simulink model "mcb_open_loop_control_nucleo_f401re"  (R2024b)
settings: Solver=FixedStepDiscrete  StartTime=0.0  StopTime=inf  RelTol=1e-3  EnableMultiTasking=on
InitFcn:
  | mcb_open_loop_control_data;
  | 
  | target.model                = 'NUCLEO-F446RE';	  % 	// Manufacturer Model Number
  | target.sn                   = 'xx';          	  % 	// Manufacturer Serial Number
  | target.CPU_frequency        = 84e6;    		  %Hz  // Clock frequency
  | target.PWM_frequency        = PWM_frequency;   	  %Hz  // PWM frequency
  | target.PWM_Counter_Period   = ...
  |  round(target.CPU_frequency/target.PWM_frequency/2); %    //PWM timer counts for up-down counter
  | target.ADC_Vref             = 3.3;			  %V   // ADC voltage reference for NUCLEO-F401RE
  | target.ADC_MaxCount         = 4095;			  %    // Max count for 12 bit ADC
  | %Read inverter logic from 'Configuration' panel on model
  | inverter.EnableLogic = eval(get_param([bdroot '/Open Loop Control/Parameters/Inverter'],'Value'));
model workspace (MAT data in the model file):
  MaxVsecuryte = 200
undefined symbols (not defined in the file or in its folder): DiscIntNeverNeededParam, motor, Ts
libraries: stmutilitieslib x4, stm32f4xxblockslib x4, simulink x3, mcbcontrolslib x3, stm32blockslib x2, hdlsllib x1, canmsglib x1
settings Model: STM32="{\"DigitalPortWrite\":{\"ID\":\"mcb_open_loop_control_nucleo_f401re:3779\"},\"PWMOutput\":{\"ID\":\"mcb_open_loop_control_nucleo_f401re:3778\"},\"HardwareInterrupt\":{\"ID\":\"mcb_open_loop_control_nucleo_f401re:3773\"},\"AnalogInput\":{\"ID\":\"mcb_open_loop_control_nucleo_f401re:3774\"},\"CANWrite\":{\"ID\":\"mcb_open_loop_control_nucleo_f401re:3906\"},\"CANRead\":{\"ID\":\"mcb_open_loop_control_nucleo_f401re:3916\"}}"  CodeVerificationMode=processor-in-the-loop (pil)  Creator=The MathWorks, Inc.  LastModifiedBy=aferreira
settings SolverCC: AlgebraicLoopSolver=TrustRegion  AutoInsertRateTranBlk=on  MaxZcPerStep=1
settings DataIOCC: SaveOutput=off  SaveTime=off  ReturnWorkspaceOutputs=off
settings OptimizationCC: DefaultUnderspecifiedDataType=single  EnhancedBackFolding=on  PassReuseOutputArgsAs=Individual arguments  ZeroExternalMemoryAtStartup=off  EfficientFloat2IntCast=on  MaxStackSize=512  OptimizeBlockOrder=speed  DifferentSizesBufferReuse=on  OptimizationCustomize=off  EfficientTunableParamExpr=on
settings DebuggingCC: MultiTaskDSMMsg=none  ParameterPrecisionLossMsg=none  ParameterTunabilityLossMsg=error  UnconnectedInputMsg=warning  UnconnectedOutputMsg=warning  UnconnectedLineMsg=warning  SubsystemReferenceDiagnosticForUnitTest=warning
settings HardwareCC: ProdBitPerPointer=32  ProdBitPerSizeT=32  ProdBitPerPtrDiffT=32  ProdLargestAtomicInteger=Long  ProdLargestAtomicFloat=Double  ProdWordSize=32  ProdLongLongMode=on  ProdHWDeviceType=ARM Compatible->ARM Cortex
settings ModelReferenceCC: EnableRefExpFcnMdlSchedulingChecks=on
settings SFSimCC: MATLABDynamicMemAlloc=off
settings RTWCC: Description=Embedded Coder  SystemTargetFile=ert.tlc  HardwareBoard=STM32F4xx Based  TemplateMakefile=ert_default_tmf  GenerateReport=on  Toolchain=GNU Tools for ARM Embedded Processors  BuildConfiguration=Faster Runs  IncludeHyperlinkInReport=on  CodeProfilingSaveOptions=AllData  GenerateTraceInfo=on  GenerateTraceReport=on  GenerateTraceReportSl=on  GenerateTraceReportSf=on  GenerateTraceReportEml=on  GPUComputeCapability=3.5  DLArmComputeVersion=19.05
settings CodeAppCC: ForceParamTrailComments=on  IgnoreCustomStorageClasses=off  OperatorAnnotations=on  SimulinkDataObjDesc=on  SFDataObjDesc=on  InsertBlockDesc=on
settings ERTTargetCC: TargetLangStandard=C99 (ISO)  CodeReplacementLibrary=ARM Cortex-M  ExtModeTransport=3  ExtModeStaticAlloc=on  ExtModeStaticAllocSize=16384  ExtModeMexFile=ext_xcp  ExtModeIntrfLevel=Level2 - Open  InlinedParameterPlacement=Hierarchical  DynamicArrayContainerType=coder::array

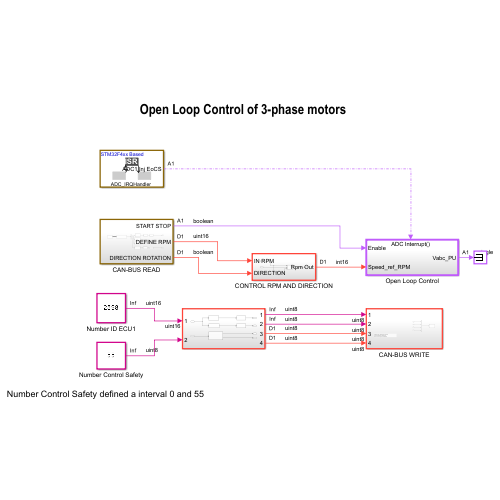
[thumbnail: Simulink's stored preview of the top-level diagram]
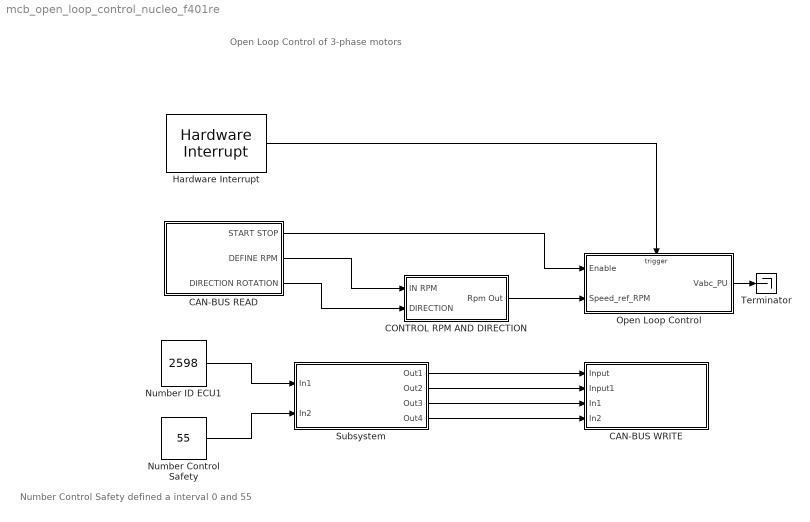
== system mcb_open_loop_control_nucleo_f401re ==
  note: Open Loop Control of 3-phase motors
  note: Number Control Safety defined a interval 0 and 55
  CAN-BUS READ : Subsystem
  CAN-BUS WRITE : Subsystem
  CONTROL RPM AND DIRECTION : Subsystem
  Hardware Interrupt : stm32f4xxblockslib/Hardware Interrupt  ISRGroup=Analog to digital converter (ADC)  ISRName=ADC_IRQHandler  ISRNumber=33  EventsList={ 'off', 'ADC1 OVR', '1'; 'off', 'ADC1 Reg EoCS', '2'; 'on', 'ADC1 Inj EoCS', '3'; 'off', 'ADC1 Watchdog', '4'; 'off', 'ADC2 OVR', '5'; 'off', 'ADC2 Reg EoCS', '6'; 'off', 'ADC2 Inj EoCS', '7'; 'off', 'ADC2 Watchdog', '8'; 'off', 'ADC3 OVR', '9'; 'off', 'ADC3 Reg EoCS', '10'; 'off', 'ADC3 Inj EoCS', '11'; 'off', 'ADC3 Watchdog', '12'; 'off', 'Custom event', '13' }  SelectedEvents={'ADC1 Inj EoCS'}  TaskPriority=30  DisablePreemption=off  ClearInterruptFlagsAtEndOfEvent=off  InterruptDefinitionFile=$(TARGET_ROOT)/registry/interrupts/STM32F4xxBased_interrupts.xml  HardwareBoard=STM32F4xx Based  EnableSimPort=off
  Number Control Safety : Constant  Value=55  OutMin=0  OutMax=55  OutDataTypeStr=uint8
  Number ID ECU1 : Constant  Value=2598  OutDataTypeStr=uint16
  Open Loop Control : Subsystem
  Subsystem : Subsystem
  Terminator : Terminator
  wires:
  Open Loop Control/1(Vabc_PU) -> Terminator/1
  Hardware Interrupt/1 -> Open Loop Control/Trigger
  CAN-BUS READ/2(DEFINE RPM) -> CONTROL RPM AND DIRECTION/1(IN RPM)
  CAN-BUS READ/3(DIRECTION ROTATION) -> CONTROL RPM AND DIRECTION/2(DIRECTION)
  CONTROL RPM AND DIRECTION/1(Rpm Out) -> Open Loop Control/2(Speed_ref_RPM)
  CAN-BUS READ/1(START STOP) -> Open Loop Control/1(Enable)
  Number ID ECU1/1 -> Subsystem/1(In1)
  Number Control Safety/1 -> Subsystem/2(In2)
  Subsystem/1(Out1) -> CAN-BUS WRITE/1(Input)
  Subsystem/2(Out2) -> CAN-BUS WRITE/2(Input1)
  Subsystem/3(Out3) -> CAN-BUS WRITE/3(In1)
  Subsystem/4(Out4) -> CAN-BUS WRITE/4(In2)

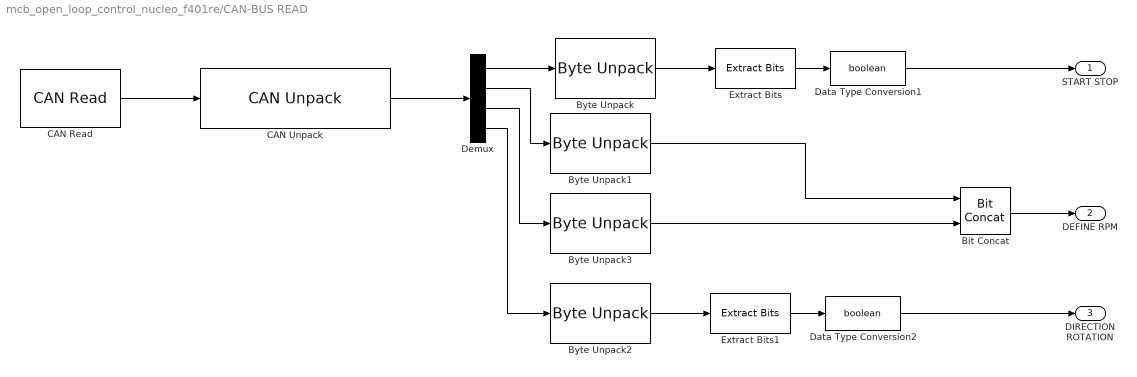
== system mcb_open_loop_control_nucleo_f401re/CAN-BUS READ ==
  Bit Concat : hdlsllib/Logic and Bit Operations/Bit Concat  numInputs=2
  Byte Unpack{,1..3} (4 alike) : stmutilitieslib/Byte Unpack  dimensions={[1]}  datatypes={'uint8'}  byteAlign=1  blockPlatform=stm32f4discovery
  CAN Read : stm32blockslib/CAN Read  CANModule=CAN1  BlockMode=Receive  OperationReadMode=Data  OperationWriteMode=Data  OutputTypeReadMode=Packed  DataFormatWriteMode=Raw data  ReadSource=FIFO 0  IdentifierTypeVia=Dialog  IdentifierType=Standard (11-bit identifier)  IdentifierVia=Inport  Identifier=100  DataLengthVia=Inport  DataLength=8  OutputIdType=off  TransmitRemoteFrame=off  OutputRemoteFrame=off  OutputTxFifoLevel=off  OutputRxFifoLevel=off  OutputStatus=off  Timeout=0.001  SampleTime=-1
      settings: LibrarySourceBlock=stm32f4xxblockslib/CAN Read
  CAN Unpack : canmsglib/CAN Unpack  MsgList=(none)  MsgName=CAN Msg  MsgIDType=Standard (11-bit identifier)  MsgIdentifier=0x220  MsgLength=4  SignalInfo={}  IDPort=off  TimestampPort=off  ErrorPort=off  RemotePort=off  LengthPort=off  StatusPort=off  ApplyMinMax=off
      settings: LibrarySourceBlock=stmutilitieslib/CAN Unpack  DataFormat=raw data
  Data Type Conversion1 : DataTypeConversion  OutDataTypeStr=boolean  SaturateOnIntegerOverflow=off  RndMeth=Floor
  Data Type Conversion2 : DataTypeConversion  OutDataTypeStr=boolean  SaturateOnIntegerOverflow=off  RndMeth=Floor
  Demux : Demux
  Extract Bits : simulink/Logic and Bit Operations/Extract Bits  bitsToExtract=Range of bits  numBits=8  bitIdxRange=[0]  outScalingMode=Preserve fixed-point scaling
  Extract Bits1 : simulink/Logic and Bit Operations/Extract Bits  bitsToExtract=Range of bits  numBits=8  bitIdxRange=[0]  outScalingMode=Preserve fixed-point scaling
  START STOP : Outport
  DEFINE RPM : Outport  Port=2
  DIRECTION ROTATION : Outport  Port=3
  wires:
  CAN Unpack/1 -> Demux/1
  Demux/1 -> Byte Unpack/1
  Data Type Conversion1/1 -> START STOP/1
  Byte Unpack/1 -> Extract Bits/1
  CAN Read/1 -> CAN Unpack/1
  Demux/2 -> Byte Unpack1/1
  Extract Bits/1 -> Data Type Conversion1/1
  Extract Bits1/1 -> Data Type Conversion2/1
  Data Type Conversion2/1 -> DIRECTION ROTATION/1
  Byte Unpack2/1 -> Extract Bits1/1
  Demux/3 -> Byte Unpack3/1
  Demux/4 -> Byte Unpack2/1
  Bit Concat/1 -> DEFINE RPM/1
  Byte Unpack1/1 -> Bit Concat/1
  Byte Unpack3/1 -> Bit Concat/2

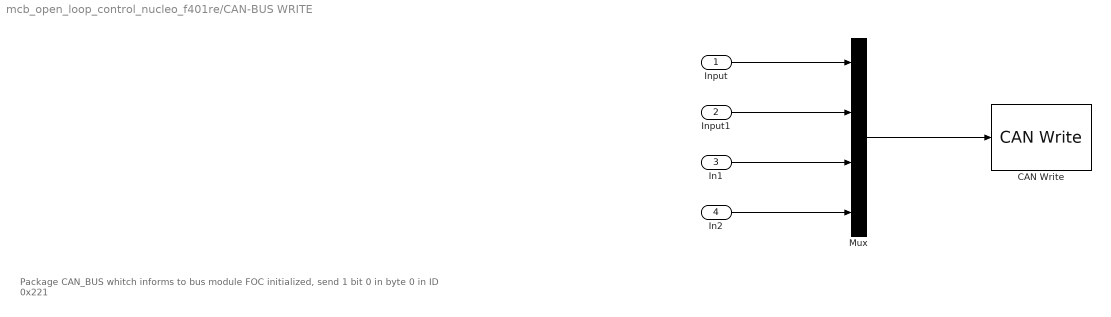
== system mcb_open_loop_control_nucleo_f401re/CAN-BUS WRITE ==
  note: Package CAN_BUS whitch informs
      | to bus module FOC initialized,
      | send 1 bit 0 in byte 0 in ID 0x221
  Input : Inport  OutDataTypeStr=uint8
  Input1 : Inport  Port=2  OutDataTypeStr=uint8
  In1 : Inport  Port=3  OutDataTypeStr=uint8
  In2 : Inport  Port=4  OutDataTypeStr=uint8
  CAN Write : stm32blockslib/CAN Write  CANModule=CAN1  BlockMode=Transmit  OperationReadMode=Data  OperationWriteMode=Data  OutputTypeReadMode=Unpacked  DataFormatWriteMode=Raw data  ReadSource=FIFO 0  IdentifierTypeVia=Dialog  IdentifierType=Standard (11-bit identifier)  IdentifierVia=Dialog  Identifier=0x221  DataLengthVia=Dialog  DataLength=4  OutputIdType=off  TransmitRemoteFrame=off  OutputRemoteFrame=off  OutputTxFifoLevel=off  OutputRxFifoLevel=off  OutputStatus=off  Timeout=0.1  SampleTime=-1
      settings: LibrarySourceBlock=stm32f4xxblockslib/CAN Write
  Mux : Mux
  wires:
  Mux/1 -> CAN Write/1
  Input/1 -> Mux/1
  Input1/1 -> Mux/2
  In1/1 -> Mux/3
  In2/1 -> Mux/4

== system mcb_open_loop_control_nucleo_f401re/CONTROL RPM AND DIRECTION ==
  IN RPM : Inport
  DIRECTION : Inport  Port=2
  Gain : Gain  Gain=-1  ParamDataTypeStr=int16  OutDataTypeStr=int16  RndMeth=Simplest
  Switch : Switch  Criteria=u2 ~= 0  OutDataTypeStr=int16  RndMeth=Simplest  SaturateOnIntegerOverflow=off  InputSameDT=off
  Rpm Out : Outport
  wires:
  Switch/1 -> Rpm Out/1
  IN RPM/1 -> Gain/1, Switch/1
  DIRECTION/1 -> Switch/2
  Gain/1 -> Switch/3

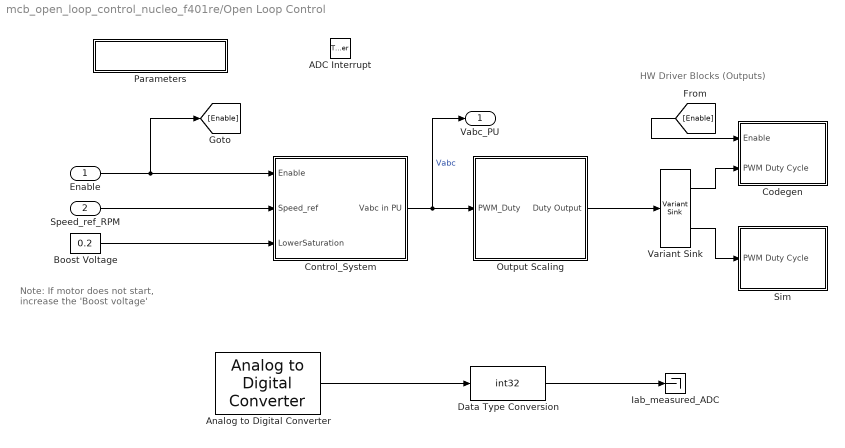
== system mcb_open_loop_control_nucleo_f401re/Open Loop Control ==
  note: Note: If motor does not start, increase the 'Boost voltage'
  note: HW Driver Blocks (Outputs)
  Enable : Inport
  Speed_ref_RPM : Inport  Port=2
  ADC Interrupt : TriggerPort  TriggerType=function-call  VariantControl=Variant
  Analog to Digital Converter : stm32f4xxblockslib/Analog to Digital Converter  ADCModule=ADC1  ConversionGroup=Injected  TriggerMode=Read results only  NumberOfConversions=2  EnableBufferConv=off  BufferLength=1  OutputStatus=off  SampleTime=-1  EnableSimPort=off  hoistedMaskSrc=ECSoC/ECSimCodegen/Analog to Digital Converter
  Boost Voltage : Constant  Value=0.2  OutDataTypeStr=dataType
  Codegen : Subsystem
      settings: RTWSystemCode=Nonreusable function
  Control_System : Subsystem
      settings: RTWSystemCode=Nonreusable function
  Data Type Conversion : DataTypeConversion  OutDataTypeStr=int32  ConvertRealWorld=Stored Integer (SI)  SaturateOnIntegerOverflow=off  RndMeth=Floor
  Iab_measured_ADC : Terminator
  Output Scaling : Subsystem
      settings: RTWSystemCode=Nonreusable function
  Parameters : Subsystem
  Sim : Subsystem
  Variant Sink : VariantSink  VariantControlMode=sim codegen switching
  Vabc_PU : Outport  VectorParamsAs1DForOutWhenUnconnected=off
  wires:
  Control_System/1(Vabc in PU) -> Output Scaling/1(PWM_Duty), Vabc_PU/1  "Vabc"
  Boost Voltage/1 -> Control_System/3(LowerSaturation)
  Data Type Conversion/1 -> Iab_measured_ADC/1
  Enable/1 -> [Enable], Control_System/1(Enable)
  Speed_ref_RPM/1 -> Control_System/2(Speed_ref)
  Analog to Digital Converter/1 -> Data Type Conversion/1
  [Enable] -> Codegen/1(Enable)
  Variant Sink/1 -> Codegen/2(PWM Duty Cycle)
  Variant Sink/2 -> Sim/1(PWM Duty Cycle)
  Output Scaling/1(Duty Output) -> Variant Sink/1

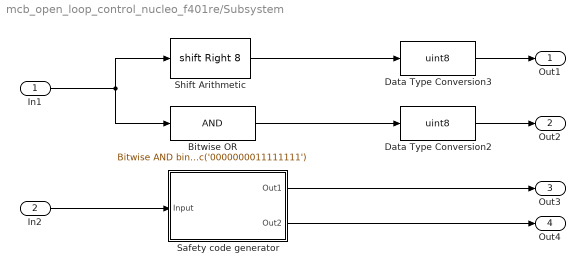
== system mcb_open_loop_control_nucleo_f401re/Subsystem ==
  In1 : Inport  OutDataTypeStr=uint16
  In2 : Inport  Port=2
  Bitwise OR : simulink/Logic and Bit Operations/Bitwise Operator  logicop=AND  UseBitMask=on  BitMask=bin2dec('0000000011111111')  BitMaskRealWorld=Stored Integer
  Data Type Conversion2 : DataTypeConversion  OutDataTypeStr=uint8  SaturateOnIntegerOverflow=off  RndMeth=Floor
  Data Type Conversion3 : DataTypeConversion  OutDataTypeStr=uint8  SaturateOnIntegerOverflow=off  RndMeth=Floor
  Safety code generator : Subsystem
  Shift Arithmetic : ArithShift  BitShiftNumber=8  BitShiftDirection=Right
  Out1 : Outport  OutDataTypeStr=uint8
  Out2 : Outport  Port=2  OutDataTypeStr=uint8
  Out3 : Outport  Port=3  OutDataTypeStr=uint8
  Out4 : Outport  Port=4  OutDataTypeStr=uint8
  wires:
  Data Type Conversion3/1 -> Out1/1
  In2/1 -> Safety code generator/1(Input)
  Data Type Conversion2/1 -> Out2/1
  Safety code generator/2(Out2) -> Out4/1
  Safety code generator/1(Out1) -> Out3/1
  Bitwise OR/1 -> Data Type Conversion2/1
  In1/1 -> Bitwise OR/1, Shift Arithmetic/1
  Shift Arithmetic/1 -> Data Type Conversion3/1

== system mcb_open_loop_control_nucleo_f401re/Open Loop Control/Codegen ==
  Enable : Inport
  PWM Duty Cycle : Inport  Port=2
  Hardware Initialization : Subsystem
      settings: RTWSystemCode=Nonreusable function
  PWM Output : Subsystem
      settings: RTWSystemCode=Nonreusable function
  wires:
  PWM Duty Cycle/1 -> PWM Output/1(PWM Duty Cycle)
  Enable/1 -> Hardware Initialization/1(Enable), PWM Output/2(Enable)

== system mcb_open_loop_control_nucleo_f401re/Open Loop Control/Control_System ==
  Enable : Inport
  Speed_ref : Inport  Port=2
  LowerSaturation : Inport  Port=3
  SpeedRefToFreq : Subsystem
  VabcCalc : Subsystem
  Vabc in PU : Outport  VectorParamsAs1DForOutWhenUnconnected=off
  wires:
  Speed_ref/1 -> SpeedRefToFreq/2(Speed_Ref)
  SpeedRefToFreq/1(Frequency) -> VabcCalc/1(Frequency)
  VabcCalc/1(Vabc) -> Vabc in PU/1
  LowerSaturation/1 -> VabcCalc/2(LowerSaturation)
  Enable/1 -> SpeedRefToFreq/1(Enable)

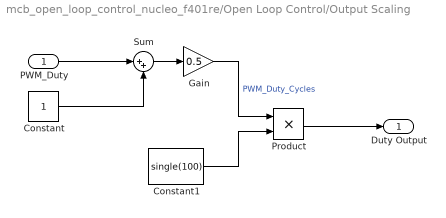
== system mcb_open_loop_control_nucleo_f401re/Open Loop Control/Output Scaling ==
  PWM_Duty : Inport
  Constant : Constant  OutDataTypeStr=dataType
  Constant1 : Constant  Value=single(100)
  Gain : Gain  Gain=0.5  RndMeth=Simplest  OutDataTypeStr=Inherit: Same as input
  Product : Product  RndMeth=Simplest  OutDataTypeStr=Inherit: Same as first input
  Sum : Sum  Inputs=|++
  Duty Output : Outport
  wires:
  Product/1 -> Duty Output/1
  Constant1/1 -> Product/2
  PWM_Duty/1 -> Sum/1
  Constant/1 -> Sum/2
  Sum/1 -> Gain/1
  Gain/1 -> Product/1  "PWM_Duty_Cycles"

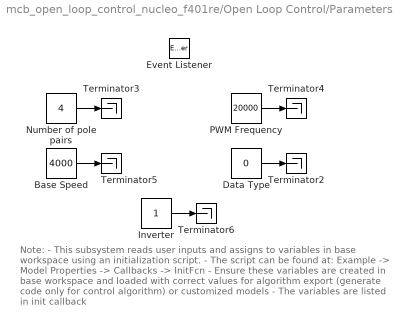
== system mcb_open_loop_control_nucleo_f401re/Open Loop Control/Parameters ==
  note: Note:
      | - This subsystem reads user inputs and assigns to variables
      | in base workspace using an initialization script.
      | - The script can be found at: Example -> Model Properties ->
      | Callbacks -> InitFcn
      | - Ensure these variables are created in base workspace and
      | loaded with correct values for algorithm export (generate
      | code only for control algorithm) or customized models
      | - The variables are listed in init callback
  Base Speed : Constant  Value=4000
  Data Type : Constant  Value=0
  Event Listener : EventListener  DisableCoverage=on  EventName=reset
  Inverter : Constant
  Number of pole pairs : Constant  Value=4
  PWM Frequency : Constant  Value=20000
  Terminator{2..6} (5 alike) : Terminator
  wires:
  Data Type/1 -> Terminator2/1
  Number of pole pairs/1 -> Terminator3/1
  PWM Frequency/1 -> Terminator4/1
  Base Speed/1 -> Terminator5/1
  Inverter/1 -> Terminator6/1

== system mcb_open_loop_control_nucleo_f401re/Open Loop Control/Sim ==
  PWM Duty Cycle : Inport
  Terminator : Terminator
  wires:
  PWM Duty Cycle/1 -> Terminator/1

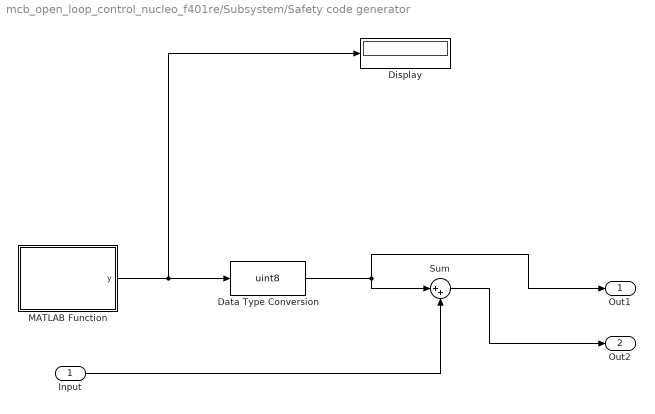
== system mcb_open_loop_control_nucleo_f401re/Subsystem/Safety code generator ==
  Input : Inport
  Data Type Conversion : DataTypeConversion  OutDataTypeStr=uint8  SaturateOnIntegerOverflow=off  RndMeth=Floor
  Display : Display
  MATLAB Function : MATLAB Function  TreatAsAtomicUnit=on
  Sum : Sum  Inputs=|++
  Out1 : Outport  OutDataTypeStr=uint8
  Out2 : Outport  Port=2  OutDataTypeStr=uint8
  wires:
  Data Type Conversion/1 -> Sum/1, Out1/1
  Input/1 -> Sum/2
  Sum/1 -> Out2/1
  MATLAB Function/1(y) -> Display/1, Data Type Conversion/1

== system mcb_open_loop_control_nucleo_f401re/Open Loop Control/Codegen/Hardware Initialization ==
  Enable : Inport
  Constant1 : Constant  Value=inverter.EnableLogic  OutDataTypeStr=uint16
  Digital Port Write : stm32f4xxblockslib/Digital Port Write  PortName=GPIOC  PinNumber=[10 11 12]  ReadOperation=off  IOAsArray=off  EnableSimPort=off  hoistedMaskSrc=ECSoC/ECSimCodegen/Digital Port Write
  NOT : Logic  Operator=NOT  IconShape=distinctive  AllPortsSameDT=off  OutDataTypeStr=boolean
  Switch : Switch  Criteria=u2 > Threshold  OutDataTypeStr=boolean  RndMeth=Simplest  SaturateOnIntegerOverflow=off  InputSameDT=off
  wires:
  Enable/1 -> NOT/1, Switch/1
  Constant1/1 -> Switch/2
  NOT/1 -> Switch/3
  Switch/1 -> Digital Port Write/3, Digital Port Write/2, Digital Port Write/1

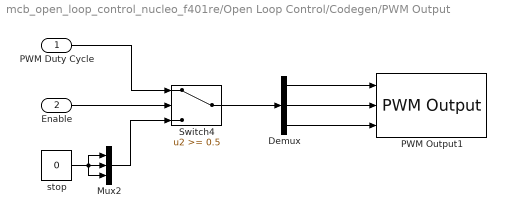
== system mcb_open_loop_control_nucleo_f401re/Open Loop Control/Codegen/PWM Output ==
  PWM Duty Cycle : Inport
  Enable : Inport  Port=2
  Demux : Demux  Outputs=3
  Mux2 : Mux  Inputs=3
  PWM Output1 : stm32f4xxblockslib/PWM Output  TimerModule=TIM1  DutycycleUnits=Percentage  EnableChannel1=on  EnableChannel2=on  EnableChannel3=on  EnableChannel4=off  EnableCounterInput=off  EnableMainOutputInput=off  EnableFrequencyInput=off  SetRCAfterCE=off  OutputDirection=off  OutputMainOutputEnableStatus=off  SampleTime=0.1  EnableSimPort=off  EnableUpdateEvent=off  EnableCaptureCompare1Event=off  EnableCaptureCompare2Event=off  EnableCaptureCompare3Event=off  EnableCaptureCompare4Event=off  EnableTriggerEvent=off  EnableBreakEvent=off  ProcessorFamily=STM32F4  hoistedMaskSrc=ECSoC/ECSimCodegen/PWM Output
  Switch4 : Switch  Threshold=0.5  RndMeth=Simplest  SaturateOnIntegerOverflow=off  InputSameDT=off
  stop : Constant  Value=0  OutDataTypeStr=single
  wires:
  Demux/3 -> PWM Output1/3
  Demux/2 -> PWM Output1/2
  PWM Duty Cycle/1 -> Switch4/1
  Demux/1 -> PWM Output1/1
  stop/1 -> Mux2/3, Mux2/2, Mux2/1
  Switch4/1 -> Demux/1
  Mux2/1 -> Switch4/3
  Enable/1 -> Switch4/2

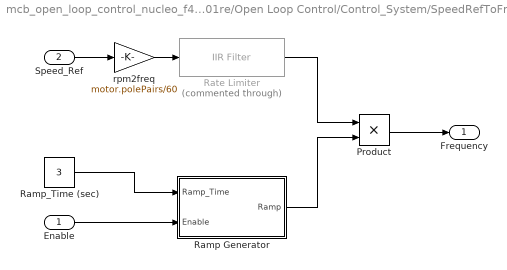
== system mcb_open_loop_control_nucleo_f401re/Open Loop Control/Control_System/SpeedRefToFreq ==
  Enable : Inport
  Speed_Ref : Inport  Port=2
  Product : Product  RndMeth=Simplest  OutDataTypeStr=Inherit: Same as first input
  Ramp Generator : Subsystem
  Ramp_Time (sec) : Constant  Value=3  OutDataTypeStr=dataType  SampleTime=-1
  Rate Limiter : mcbcontrolslib/IIR Filter  Commented=through  VariantControl=Low Pass Filter  VariantSelect=Low-pass  FilterConstantInputType=Specify via dialog  Filter_constant=0.0001  advancedSettings=off  Ts=50e-6  cutOff_freq=0.31834
  rpm2freq : Gain  Gain=motor.polePairs/60  OutDataTypeStr=dataType  RndMeth=Simplest
  Frequency : Outport
  wires:
  Product/1 -> Frequency/1
  Ramp Generator/1(Ramp) -> Product/2
  Ramp_Time (sec)/1 -> Ramp Generator/1(Ramp_Time)
  rpm2freq/1 -> Rate Limiter/1
  Enable/1 -> Ramp Generator/2(Enable)
  Speed_Ref/1 -> rpm2freq/1
  Rate Limiter/1 -> Product/1

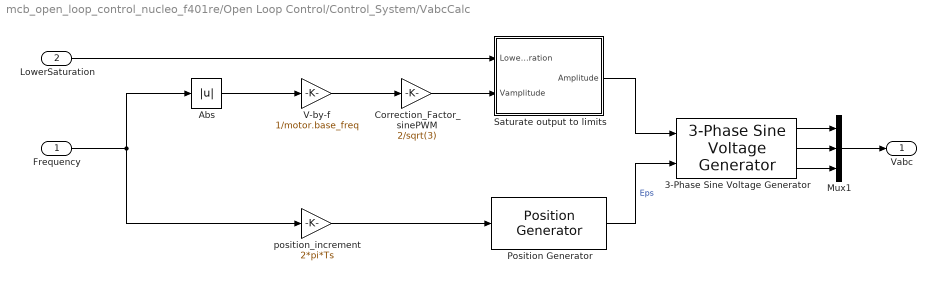
== system mcb_open_loop_control_nucleo_f401re/Open Loop Control/Control_System/VabcCalc ==
  Frequency : Inport
  LowerSaturation : Inport  Port=2
  3-Phase Sine Voltage Generator : mcbcontrolslib/3-Phase Sine Voltage Generator  AngleInput=Radians  N_points=1024
  Abs : Abs  RndMeth=Simplest  SaturateOnIntegerOverflow=off
  Correction_Factor_sinePWM : Gain  Gain=2/sqrt(3)  RndMeth=Simplest  OutDataTypeStr=Inherit: Same as input
  Mux1 : Mux  Inputs=3
  Position Generator : mcbcontrolslib/Position Generator  AngleOutput=Radians  ExternalReset=none  Offset=0
  Saturate output to limits : Subsystem
  V-by-f : Gain  Gain=1/motor.base_freq  RndMeth=Simplest  OutDataTypeStr=Inherit: Same as input
  position_increment : Gain  Gain=2*pi*Ts  RndMeth=Simplest  OutDataTypeStr=Inherit: Same as input
  Vabc : Outport
  wires:
  Frequency/1 -> Abs/1, position_increment/1
  position_increment/1 -> Position Generator/1
  3-Phase Sine Voltage Generator/3 -> Mux1/3
  3-Phase Sine Voltage Generator/2 -> Mux1/2
  V-by-f/1 -> Correction_Factor_sinePWM/1
  3-Phase Sine Voltage Generator/1 -> Mux1/1
  Correction_Factor_sinePWM/1 -> Saturate output to limits/2(Vamplitude)
  Mux1/1 -> Vabc/1
  LowerSaturation/1 -> Saturate output to limits/1(Lower Saturation)
  Saturate output to limits/1(Amplitude) -> 3-Phase Sine Voltage Generator/1
  Position Generator/1 -> 3-Phase Sine Voltage Generator/2  "Eps"
  Abs/1 -> V-by-f/1

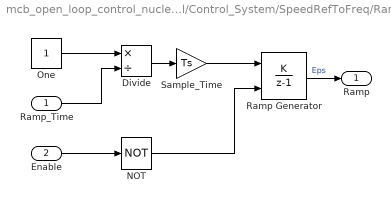
== system mcb_open_loop_control_nucleo_f401re/Open Loop Control/Control_System/SpeedRefToFreq/Ramp Generator ==
  Ramp_Time : Inport
  Enable : Inport  Port=2
  Divide : Product  Inputs=*/  RndMeth=Simplest  OutDataTypeStr=Inherit: Same as first input
  NOT : Logic  Operator=NOT  IconShape=distinctive  AllPortsSameDT=off  OutDataTypeStr=boolean
  One : Constant  OutDataTypeStr=dataType  SampleTime=-1
  Ramp Generator : DiscreteIntegrator  IntegratorMethod=Accumulation: Forward Euler  gainval=1  ExternalReset=sampled level  SampleTime=-1  OutDataTypeStr=dataType  RndMeth=Simplest  LimitOutput=on  UpperSaturationLimit=1  LowerSaturationLimit=0  ICPrevOutput=DiscIntNeverNeededParam  ICPrevScaledInput=DiscIntNeverNeededParam
  Sample_Time : Gain  Gain=Ts  RndMeth=Simplest  OutDataTypeStr=Inherit: Same as input
  Ramp : Outport
  wires:
  Divide/1 -> Sample_Time/1
  Ramp Generator/1 -> Ramp/1  "Eps"
  Sample_Time/1 -> Ramp Generator/1
  One/1 -> Divide/1
  Ramp_Time/1 -> Divide/2
  Enable/1 -> NOT/1
  NOT/1 -> Ramp Generator/2

== system mcb_open_loop_control_nucleo_f401re/Open Loop Control/Control_System/VabcCalc/Saturate output to limits ==
  Lower Saturation : Inport
  Vamplitude : Inport  Port=2
  Relational Operator : RelationalOperator  Operator=>  OutDataTypeStr=boolean  RndMeth=Simplest  InputSameDT=off
  Saturation : Saturate  UpperLimit=0.95  LowerLimit=0  RndMeth=Simplest
  Switch : Switch  Criteria=u2 > Threshold  SaturateOnIntegerOverflow=off  InputSameDT=off
  Amplitude : Outport
  wires:
  Saturation/1 -> Amplitude/1
  Switch/1 -> Saturation/1
  Relational Operator/1 -> Switch/2
  Lower Saturation/1 -> Switch/3, Relational Operator/2
  Vamplitude/1 -> Switch/1, Relational Operator/1

== matlab function mcb_open_loop_control_nucleo_f401re/Subsystem/Safety code generator/MATLAB Function ==
  data: y output
function y = random_on_start()
    persistent r;
    if isempty(r)
    rng('shuffle');
    r = randi([0, 200]);
end
y = r;
end
